simulink model "Quaternions_Method_merge_1"  (R2021b)
settings: Solver=VariableStepAuto  StartTime=0.0  StopTime=Time  FixedStep=1e-3  MinStep=1e-3  RelTol=1e-13  AbsTol=1e-8
values from neighbouring files (symbols this model uses):
  a = 8.6251e+06    (= 8625100)    [Main.m]
  c = 299792*10^3    (= 299792000)    [Main.m]
  e = 0.1195    [Main.m]
  f_mag = 5    [Main.m]
  H_0 = sqrt((g_1_0)^2 + (g_1_1)^2 + (h_1_1)^2)    [Main.m]
  i = 0.3815    [Main.m]
  MB = [2000; 0.3; 1; 0.12].*1e-2    [Main.m]
  mr = 1.2 * 0.0001    (= 0.00012)    [Main.m]
  muP = G*Mt    (= 398527110340000)    [Main.m]
  omega_0 = [om_x, om_y, om_z]    [Main.m]
  p_acc = deg2rad(5)    [Main.m]
  RD = 0.1*ones(1,10)    [Main.m]
  RS_MB = 0.5    [Main.m]
  RS_SP = 0.1    [Main.m]
  SP = [2000; 0.3; 1; 0.12].*1e-2    [Main.m]
  theta0 = 0    [Main.m]
  w_E = (2*pi)/(24*3600)    (= 7.27220521664e-05)    [Main.m]
undefined symbols (not defined in the file or in its folder): magnitude
libraries: matrix_library x10, vrlib x5, simulink_extras x1, simulink x1
(part 2 of 3)

== system Quaternions_Method_merge_1/Kinematics/Creazione Matrice A_BN/column 2 ==
  q_normalizzato : Inport
  Demux : Demux
  Gain : Gain  Gain=2
  Gain1 : Gain  Gain=2
  Mux : Mux  Inputs=3
  Product{,1..3} (4 alike) : Product
  Square{,1..3} (4 alike) : Math  Operator=square  SaturateOnIntegerOverflow=on
  Sum : Sum  Inputs=|-|+|-|+|
  Sum1 : Sum  Inputs=|+|+|
  Sum2 : Sum  Inputs=|+|-|
  Column 2 : Outport
  wires:
  Demux/4 -> [q4]
  Demux/1 -> [q1]
  q_normalizzato/1 -> Demux/1
  Demux/3 -> [q3]
  Demux/2 -> [q2]
  Mux/1 -> Column 2/1
  Gain1/1 -> Mux/3
  Product2/1 -> Sum2/1
  Product3/1 -> Sum2/2
  Sum2/1 -> Gain1/1
  Sum1/1 -> Gain/1
  [q2] -> Product/2
  [q3] -> Product1/1
  [q4] -> Product1/2
  Product/1 -> Sum1/1
  Gain/1 -> Mux/1
  [q1] -> Product/1
  Product1/1 -> Sum1/2
  Sum/1 -> Mux/2
  [q1] -> Square/1
  Square1/1 -> Sum/4
  Square3/1 -> Sum/2
  [q4] -> Square1/1
  Square2/1 -> Sum/3
  [q2] -> Square3/1
  [q3] -> Square2/1
  Square/1 -> Sum/1
  [q2] -> Product2/1
  [q3] -> Product2/2
  [q1] -> Product3/1
  [q4] -> Product3/2

== system Quaternions_Method_merge_1/Kinematics/Creazione Matrice A_BN/column 3 ==
  q_normalizzato : Inport
  Demux : Demux
  Gain : Gain  Gain=2
  Gain1 : Gain  Gain=2
  Mux : Mux  Inputs=3
  Product{,1..3} (4 alike) : Product
  Square{,1..3} (4 alike) : Math  Operator=square  SaturateOnIntegerOverflow=on
  Sum : Sum  Inputs=|-|-|+|+|
  Sum1 : Sum  Inputs=|+|-|
  Sum2 : Sum  Inputs=|+|+|
  Column 3 : Outport
  wires:
  Demux/4 -> [q4]
  Demux/1 -> [q1]
  q_normalizzato/1 -> Demux/1
  Demux/3 -> [q3]
  Demux/2 -> [q2]
  Gain/1 -> Mux/1
  Product1/1 -> Sum1/2
  [q4] -> Product1/2
  Product/1 -> Sum1/1
  Mux/1 -> Column 3/1
  [q1] -> Product/1
  Sum1/1 -> Gain/1
  [q1] -> Square/1
  Square2/1 -> Sum/3
  Square3/1 -> Sum/2
  [q4] -> Square1/1
  Square1/1 -> Sum/4
  Square/1 -> Sum/1
  Sum/1 -> Mux/3
  [q3] -> Square2/1
  [q2] -> Square3/1
  [q2] -> Product2/1
  Product3/1 -> Sum2/2
  Gain1/1 -> Mux/2
  Sum2/1 -> Gain1/1
  Product2/1 -> Sum2/1
  [q3] -> Product2/2
  [q4] -> Product3/2
  [q1] -> Product3/1
  [q3] -> Product/2
  [q2] -> Product1/1

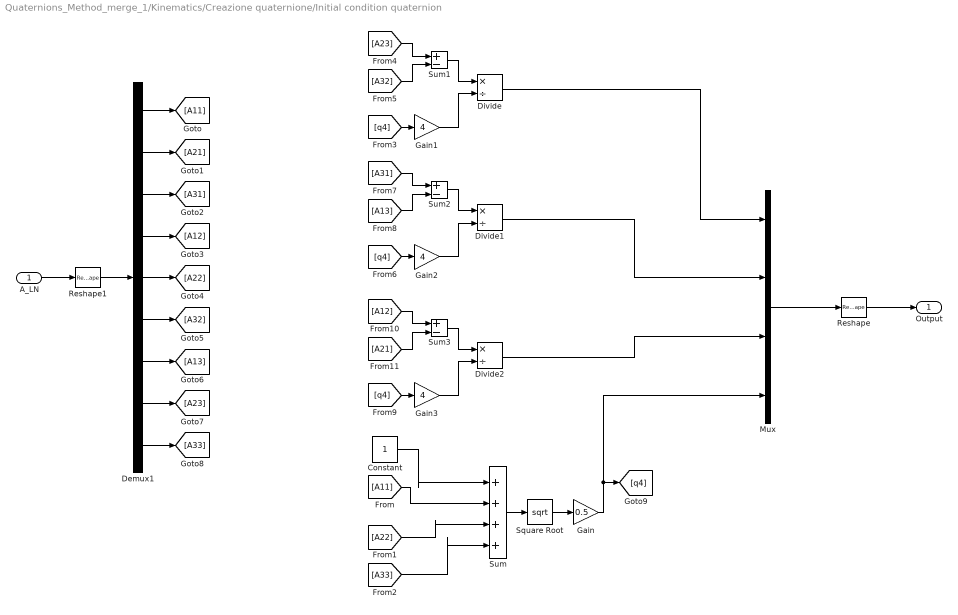
== system Quaternions_Method_merge_1/Kinematics/Creazione quaternione/Initial condition quaternion ==
  A_LN : Inport
  Constant : Constant
  Demux1 : Demux  Outputs=9
  Divide : Product  Inputs=*/
  Divide1 : Product  Inputs=*/
  Divide2 : Product  Inputs=*/
  Gain : Gain  Gain=0.5
  Gain1 : Gain  Gain=4
  Gain2 : Gain  Gain=4
  Gain3 : Gain  Gain=4
  Mux : Mux
  Reshape : Reshape  OutputDimensionality=Column vector (2-D)
  Reshape1 : Reshape  OutputDimensionality=Column vector (2-D)
  Square Root : Sqrt  SaturateOnIntegerOverflow=on
  Sum : Sum  Inputs=|+|+|+|+|
  Sum1 : Sum  Inputs=|+|-|
  Sum2 : Sum  Inputs=|+|-|
  Sum3 : Sum  Inputs=|+|-|
  Output : Outport
  wires:
  Demux1/3 -> [A31]
  Demux1/9 -> [A33]
  Demux1/1 -> [A11]
  A_LN/1 -> Reshape1/1
  Reshape1/1 -> Demux1/1
  Demux1/5 -> [A22]
  Demux1/2 -> [A21]
  Demux1/4 -> [A12]
  Demux1/6 -> [A32]
  Demux1/7 -> [A13]
  Demux1/8 -> [A23]
  Constant/1 -> Sum/1
  [A11] -> Sum/2
  [A22] -> Sum/3
  [A33] -> Sum/4
  Sum/1 -> Square Root/1
  Square Root/1 -> Gain/1
  Gain/1 -> Mux/4, [q4]
  [A23] -> Sum1/1
  [A32] -> Sum1/2
  Sum1/1 -> Divide/1
  [q4] -> Gain1/1
  Gain1/1 -> Divide/2
  Divide/1 -> Mux/1
  Divide1/1 -> Mux/2
  [A31] -> Sum2/1
  [A13] -> Sum2/2
  Sum2/1 -> Divide1/1
  [q4] -> Gain2/1
  Gain2/1 -> Divide1/2
  Divide2/1 -> Mux/3
  [A12] -> Sum3/1
  [A21] -> Sum3/2
  Sum3/1 -> Divide2/1
  [q4] -> Gain3/1
  Gain3/1 -> Divide2/2
  Mux/1 -> Reshape/1
  Reshape/1 -> Output/1

== system Quaternions_Method_merge_1/Kinematics/Creazione quaternione/Normalisation ==
  In1 : Inport
  Normalize Vector : vrlib/Utilities/Normalize Vector  maxzero=0
  Reshape : Reshape  OutputDimensionality=Column vector (2-D)
  Out1 : Outport
  wires:
  In1/1 -> Normalize Vector/1
  Normalize Vector/1 -> Reshape/1
  Reshape/1 -> Out1/1

== system Quaternions_Method_merge_1/Kinematics/Relative_Attitude/A_LN ==
  theta : Inport
  Constant : Constant  Value=i
  M1 : Subsystem
  M2 : Subsystem
  MatrixMultiply : Product  Multiplication=Matrix(*)
  A_LN : Outport
  wires:
  theta/1 -> M1/1(Input)
  M1/1(Out1) -> MatrixMultiply/1
  M2/1(Out1) -> MatrixMultiply/2
  MatrixMultiply/1 -> A_LN/1
  Constant/1 -> M2/1(ii)

== system Quaternions_Method_merge_1/Kinematics/Relative_Attitude/Orbit Propagation ==
  A_BN : Inport
  Constant : Constant  Value=muP
  Constant1 : Constant  Value=e^2
  Constant2 : Constant
  Constant3 : Constant  Value=3
  Constant4 : Constant
  Constant5 : Constant  Value=3/2
  Cos : Trigonometry  Operator=cos
  Divide : Product  Inputs=*/
  Divide1 : Product  Inputs=*/
  Divide2 : Product  Inputs=*/
  Gain : Gain  Gain=a
  Gain1 : Gain  Gain=e
  Integrator : Integrator  InitialCondition=theta0
  MatrixMultiply : Product  Multiplication=Matrix(*)
  Product : Product
  Product1 : Product
  Sqrt : Sqrt  SaturateOnIntegerOverflow=on
  Square : Math  Operator=pow  SaturateOnIntegerOverflow=on
  Square1 : Math  Operator=square  SaturateOnIntegerOverflow=on
  Square2 : Math  Operator=pow  SaturateOnIntegerOverflow=on
  Sum : Sum  Inputs=+-
  Sum1 : Sum
  vector : Subsystem
  n : Outport
  theta : Outport  Port=2
  rB : Outport  Port=3
  wires:
  Constant2/1 -> Sum/1
  Constant1/1 -> Sum/2
  Sum/1 -> Square2/1, Gain/1
  Gain/1 -> Divide/1
  Constant4/1 -> Sum1/1
  Sum1/1 -> Square1/1, Divide/2
  Gain1/1 -> Sum1/2
  Cos/1 -> Gain1/1
  Integrator/1 -> Cos/1, theta/1, vector/1(theta)  "theta"
  Divide1/1 -> Sqrt/1
  Constant/1 -> Divide1/1
  Square/1 -> Divide1/2
  Divide/1 -> Product1/1, Square/1  "R"
  Constant3/1 -> Square/2
  Sqrt/1 -> Product/1, n/1  "n"
  Square1/1 -> Product/2
  Constant5/1 -> Square2/2
  Product/1 -> Divide2/1
  Divide2/1 -> Integrator/1  "theta_dot"
  vector/1(Vector) -> Product1/2
  A_BN/1 -> MatrixMultiply/1
  Product1/1 -> MatrixMultiply/2  "rN"
  MatrixMultiply/1 -> rB/1  "rB"
  Square2/1 -> Divide2/2

== system Quaternions_Method_merge_1/Magnetometer/Magnetometer /Error Matrices ==
  A_NonOrtho : Subsystem
  A_ScaleFactor : Subsystem
  A_eps : Subsystem
  A_no : Outport
  A_sf : Outport  Port=2
  A_noise : Outport  Port=3
  wires:
  A_NonOrtho/1(A_no) -> A_no/1
  A_ScaleFactor/1(A_sf) -> A_sf/1
  A_eps/1(A_eps) -> A_noise/1

== system Quaternions_Method_merge_1/Magnetometer/Magnetometer /RC Low Pass FIlter ==
  A* : Inport
  Add : Sum  Inputs=||+||-||
  Discrete Derivative : simulink/Discrete/Discrete Derivative  gainval=10  ICPrevScaledInput=0.0  OutMin=[]  OutMax=[]  OutDataType=fixdt(1, 16)  OutScaling=2^-10  DoSatur=off
  A*_filtered : Outport
  wires:
  A*/1 -> Add/1
  Add/1 -> Discrete Derivative/1, A*_filtered/1
  Discrete Derivative/1 -> Add/2

== system Quaternions_Method_merge_1/Magnetometer/Magnetometer /orthonormalization step 1 ==
  A*(t) : Inport
  Gain : Gain  Gain=3/2
  Gain1 : Gain  Gain=1/2
  Matrix Multiply : Product  Inputs=3  Multiplication=Matrix(*)
  Sum : Sum  Inputs=-+
  Transpose : Math  Operator=transpose  SaturateOnIntegerOverflow=on
  A_BN*_filtered : Outport
  wires:
  A*(t)/1 -> Transpose/1, Gain1/1, Matrix Multiply/1, Gain/1
  Sum/1 -> A_BN*_filtered/1
  Gain/1 -> Sum/2
  Transpose/1 -> Matrix Multiply/2
  Gain1/1 -> Matrix Multiply/3
  Matrix Multiply/1 -> Sum/1

== system Quaternions_Method_merge_1/Magnetometer/Magnetometer /orthonormalization step 2 ==
  A*(t) : Inport
  Gain : Gain  Gain=3/2
  Gain1 : Gain  Gain=1/2
  Matrix Multiply : Product  Inputs=3  Multiplication=Matrix(*)
  Sum : Sum  Inputs=-+
  Transpose : Math  Operator=transpose  SaturateOnIntegerOverflow=on
  A_BN*_filtered : Outport
  wires:
  Matrix Multiply/1 -> Sum/1
  Gain1/1 -> Matrix Multiply/3
  Transpose/1 -> Matrix Multiply/2
  Gain/1 -> Sum/2
  Sum/1 -> A_BN*_filtered/1
  A*(t)/1 -> Gain/1, Matrix Multiply/1, Gain1/1, Transpose/1

== system Quaternions_Method_merge_1/Magnetometer/Magnetometer /orthonormalization step 3 ==
  A*(t) : Inport
  Gain : Gain  Gain=3/2
  Gain1 : Gain  Gain=1/2
  Matrix Multiply : Product  Inputs=3  Multiplication=Matrix(*)
  Sum : Sum  Inputs=-+
  Transpose : Math  Operator=transpose  SaturateOnIntegerOverflow=on
  A_BN*_filtered : Outport
  wires:
  A*(t)/1 -> Transpose/1, Gain1/1, Matrix Multiply/1, Gain/1
  Sum/1 -> A_BN*_filtered/1
  Gain/1 -> Sum/2
  Transpose/1 -> Matrix Multiply/2
  Gain1/1 -> Matrix Multiply/3
  Matrix Multiply/1 -> Sum/1

== system Quaternions_Method_merge_1/Magnetometer/b_B computation/Saturation ==
  b_B : Inport
  Constant : Constant  Value=mr
  Dot Product : DotProduct  InputSameDT=on  OutDataTypeStr=Inherit: Inherit via internal rule
  If : If  NumInputs=2  IfExpression=u1 < mr
  If Action Subsystem : Subsystem  TreatAsAtomicUnit=on
  If Action Subsystem1 : Subsystem  TreatAsAtomicUnit=on
  Merge : Merge
  Square Root : Sqrt  SaturateOnIntegerOverflow=on
  b_B saturated : Outport
  wires:
  b_B/1 -> If Action Subsystem1/2(In2), If Action Subsystem/1(In1), Dot Product/2, Dot Product/1
  Dot Product/1 -> Square Root/1
  If Action Subsystem/1(b_B) -> Merge/1
  If/1 -> If Action Subsystem/Action
  If Action Subsystem1/1(Out1) -> Merge/2
  If/2 -> If Action Subsystem1/Action
  Square Root/1 -> If/1
  Constant/1 -> If Action Subsystem1/1(In1), If/2
  Merge/1 -> b_B saturated/1

== system Quaternions_Method_merge_1/Enviroment/Magnetic torque /Magnetic torque in body frame/Definition of m vector ==
  Clock : Clock
  Constant : Constant  Value=eps
  Constant1 : Constant  Value=w_E
  Mux : Mux  Inputs=3
  Product : Product
  Product1 : Product
  Product2 : Product
  Reshape : Reshape  OutputDimensionality=Column vector (2-D)
  Trigonometric Function : Trigonometry
  Trigonometric Function1 : Trigonometry  Operator=cos
  Trigonometric Function2 : Trigonometry  Operator=cos
  Trigonometric Function3 : Trigonometry
  m_vect : Outport
  wires:
  Constant1/1 -> Product/1
  Clock/1 -> Product/2
  Constant/1 -> Trigonometric Function2/1, Trigonometric Function/1
  Product/1 -> Trigonometric Function3/1, Trigonometric Function1/1
  Trigonometric Function/1 -> Product2/1, Product1/1
  Trigonometric Function1/1 -> Product1/2
  Trigonometric Function3/1 -> Product2/2
  Product1/1 -> Mux/1
  Product2/1 -> Mux/2
  Trigonometric Function2/1 -> Mux/3
  Mux/1 -> Reshape/1
  Reshape/1 -> m_vect/1

== system Quaternions_Method_merge_1/Enviroment/Solar Radiation Perturbation/Force/creation of the areas of the S//C ==
  note: creation of areas of MB:
      | a=lato corto su asse x del BF; b=lato lungo lungo asse y del BF; h = spessore lungo asse z del BF
  MB : Inport
  Demux : Demux
  Product1 : Product
  Product2 : Product
  Product4 : Product
  Terminator : Terminator
  a*b_1 : Outport
  a*b_2 : Outport  Port=2
  a*h_1 : Outport  Port=3
  a*h_2 : Outport  Port=4
  b*h_1 : Outport  Port=5
  b*h_2 : Outport  Port=6
  wires:
  Demux/4 -> Product4/1, Product2/2
  Demux/3 -> Product1/2, Product4/2
  Demux/2 -> Product1/1, Product2/1
  Product1/1 -> a*b_2/1, a*b_1/1  "a*b"
  Product2/1 -> a*h_1/1, a*h_2/1  "a*h"
  Product4/1 -> b*h_2/1, b*h_1/1  "b*h"
  MB/1 -> Demux/1
  Demux/1 -> Terminator/1

== system Quaternions_Method_merge_1/Enviroment/Solar Radiation Perturbation/Sum forces/determine highlighted area ==
  note: matrice che ha per colonne i vettori distanza tra il CM del MB e i centri geom delle aree illuminate dal sole
  MB : Inport
  A_MB : Inport  Port=2
  prodscal_MB(tra norm e sun direction) : Inport  Port=3
  Demux1 : Demux  Outputs=6
  Demux2 : Demux  Outputs=6
  If : If  NumInputs=2  IfExpression=u1>0  ElseIfExpressions=u2>0
  If Action Subsystem : Subsystem  TreatAsAtomicUnit=on
  If Action Subsystem1 : Subsystem  TreatAsAtomicUnit=on
  If Action Subsystem2 : Subsystem  TreatAsAtomicUnit=on
  If Action Subsystem3 : Subsystem  TreatAsAtomicUnit=on
  If Action Subsystem4 : Subsystem  TreatAsAtomicUnit=on
  If Action Subsystem5 : Subsystem  TreatAsAtomicUnit=on
  If Action Subsystem6 : Subsystem  TreatAsAtomicUnit=on
  If Action Subsystem7 : Subsystem  TreatAsAtomicUnit=on
  If Action Subsystem8 : Subsystem  TreatAsAtomicUnit=on
  If1 : If  NumInputs=2  IfExpression=u1>0  ElseIfExpressions=u2>0
  If2 : If  NumInputs=2  IfExpression=u1>0  ElseIfExpressions=u2>0
  Merge : Merge  Inputs=3
  Merge1 : Merge  Inputs=3
  Merge2 : Merge  Inputs=3
  Mux : Mux  Inputs=3
  Product{10..15} (6 alike) : Product
  Reshape : Reshape  OutputDimensionality=Column vector (2-D)
  Reshape1 : Reshape  OutputDimensionality=Column vector (2-D)
  "creazione della matrice che ha per colonne i vettori distanza tra il CM del MB e i centri geom delle aree illuminate dal sole " : Subsystem
  distance matrix : Outport
  wires:
  Reshape/1 -> Demux2/1
  prodscal_MB(tra norm e sun direction)/1 -> Reshape/1
  Demux2/1 -> Product15/2  "x"
  Demux2/2 -> Product13/2  "y"
  Demux2/3 -> Product12/2  "z"
  Demux2/4 -> Product11/2  "-x"
  Demux2/5 -> Product10/2  "-y"
  Demux2/6 -> Product14/2  "-z"
  Demux1/1 -> Product12/1
  Mux/1 -> Reshape1/1
  Product15/1 -> If Action Subsystem/1(In1), If/1  "x"
  If/1 -> If Action Subsystem/Action
  Reshape1/1 -> "creazione della matrice che ha per colonne i vettori distanza tra il CM del MB e i centri geom delle aree illuminate dal sole "/2(A_vect)  "Areas_vect = vettore contenente le aree nelle direzioni x, y, z, -x, -y, -z"
  "creazione della matrice che ha per colonne i vettori distanza tra il CM del MB e i centri geom delle aree illuminate dal sole "/1(distance matrix) -> distance matrix/1
  A_MB/1 -> Demux1/1
  Demux1/2 -> Product14/1
  Demux1/3 -> Product13/1
  Demux1/4 -> Product10/1
  Demux1/5 -> Product15/1
  Demux1/6 -> Product11/1
  If/2 -> If Action Subsystem1/Action
  Product11/1 -> If Action Subsystem1/1(In1), If/2  "-x"
  If1/2 -> If Action Subsystem4/Action
  If1/3 -> If Action Subsystem5/Action
  If1/1 -> If Action Subsystem3/Action
  Product10/1 -> If Action Subsystem4/1(In1), If1/2  "-y"
  Product13/1 -> If Action Subsystem3/1(In1), If1/1  "y"
  If2/2 -> If Action Subsystem7/Action
  If2/3 -> If Action Subsystem8/Action
  If2/1 -> If Action Subsystem6/Action
  Product12/1 -> If Action Subsystem6/1(In1), If2/1  "z"
  Product14/1 -> If Action Subsystem7/1(In1), If2/2  "-z"
  Merge/1 -> Mux/2
  Merge2/1 -> Mux/3
  Merge1/1 -> Mux/1
  If Action Subsystem8/1(Out1) -> Merge2/3
  If Action Subsystem7/1(Out1) -> Merge2/2
  If Action Subsystem6/1(Out1) -> Merge2/1
  If Action Subsystem5/1(Out1) -> Merge/3
  If Action Subsystem4/1(Out1) -> Merge/2
  MB/1 -> "creazione della matrice che ha per colonne i vettori distanza tra il CM del MB e i centri geom delle aree illuminate dal sole "/1(MB)
  If Action Subsystem/1(Out1) -> Merge1/1
  If Action Subsystem1/1(Out1) -> Merge1/2
  If/3 -> If Action Subsystem2/Action
  If Action Subsystem2/1(Out1) -> Merge1/3
  If Action Subsystem3/1(Out1) -> Merge/1

== system Quaternions_Method_merge_1/Enviroment/Solar Radiation Perturbation/Sum forces/determine highlighted area1 ==
  prodscal_SP(tra norm e sun direction) : Inport
  Demux2 : Demux
  If : If  NumInputs=2  IfExpression=u1>0  ElseIfExpressions=u2>0
  If Action Subsystem : Subsystem  TreatAsAtomicUnit=on
  If Action Subsystem1 : Subsystem  TreatAsAtomicUnit=on
  If Action Subsystem2 : Subsystem  TreatAsAtomicUnit=on
  If Action Subsystem3 : Subsystem  TreatAsAtomicUnit=on
  If Action Subsystem4 : Subsystem  TreatAsAtomicUnit=on
  If Action Subsystem5 : Subsystem  TreatAsAtomicUnit=on
  If1 : If  NumInputs=2  IfExpression=u1>0  ElseIfExpressions=u2>0
  Merge : Merge  Inputs=3
  Merge1 : Merge  Inputs=3
  Mux : Mux  Inputs=2
  Reshape : Reshape  OutputDimensionality=Column vector (2-D)
  Reshape1 : Reshape  OutputDimensionality=Column vector (2-D)
  face illuminated : Outport
  wires:
  If Action Subsystem2/1(Out1) -> Merge/3
  If/3 -> If Action Subsystem2/Action
  Merge/1 -> Mux/1
  Demux2/1 -> If/1  "y_1"
  Mux/1 -> Reshape1/1
  Demux2/2 -> If/2  "-y_1"
  prodscal_SP(tra norm e sun direction)/1 -> Reshape/1
  Reshape/1 -> Demux2/1
  Demux2/3 -> If1/1  "y_2"
  Demux2/4 -> If1/2  "-y_2"
  Merge1/1 -> Mux/2
  Reshape1/1 -> face illuminated/1
  If/1 -> If Action Subsystem/Action
  If Action Subsystem/1(Out1) -> Merge/1
  If/2 -> If Action Subsystem1/Action
  If Action Subsystem1/1(Out1) -> Merge/2
  If Action Subsystem4/1(Out1) -> Merge1/2
  If1/2 -> If Action Subsystem4/Action
  If1/1 -> If Action Subsystem3/Action
  If1/3 -> If Action Subsystem5/Action
  If Action Subsystem5/1(Out1) -> Merge1/3
  If Action Subsystem3/1(Out1) -> Merge1/1

== system Quaternions_Method_merge_1/Kinematics/Relative_Attitude/A_LN/M1 ==
  Input : Inport
  Constant{1..2,4..5} (4 alike) : Constant  Value=0
  Constant3 : Constant
  Cos : Trigonometry  Operator=cos
  Cos1 : Trigonometry
  Cos2 : Trigonometry  Operator=cos
  Cos3 : Trigonometry
  Matrix Concatenate : Concatenate  NumInputs=3  Mode=Multidimensional array  ConcatenateDimension=2
  Multiply : Gain  Gain=-1
  Mux : Mux  Inputs=3
  Mux1 : Mux  Inputs=3
  Mux2 : Mux  Inputs=3
  Reshape : Reshape  OutputDimensionality=Column vector (2-D)
  Reshape1 : Reshape  OutputDimensionality=Column vector (2-D)
  Reshape2 : Reshape  OutputDimensionality=Column vector (2-D)
  Out1 : Outport
  wires:
  Multiply/1 -> Mux/2
  Cos/1 -> Mux/1
  Constant1/1 -> Mux/3
  Constant2/1 -> Mux1/3
  Input/1 -> Cos/1, Cos1/1, Cos3/1, Cos2/1
  Matrix Concatenate/1 -> Out1/1
  Cos3/1 -> Mux1/1
  Constant5/1 -> Mux2/1
  Cos2/1 -> Mux1/2
  Constant3/1 -> Mux2/3
  Constant4/1 -> Mux2/2
  Cos1/1 -> Multiply/1
  Mux/1 -> Reshape/1
  Reshape/1 -> Matrix Concatenate/1
  Reshape1/1 -> Matrix Concatenate/2
  Mux1/1 -> Reshape1/1
  Mux2/1 -> Reshape2/1
  Reshape2/1 -> Matrix Concatenate/3

== system Quaternions_Method_merge_1/Kinematics/Relative_Attitude/A_LN/M2 ==
  ii : Inport
  Constant{1..4} (4 alike) : Constant  Value=0
  Constant5 : Constant
  Cos : Trigonometry  Operator=cos
  Cos1 : Trigonometry
  Cos2 : Trigonometry  Operator=cos
  Cos3 : Trigonometry
  Matrix Concatenate : Concatenate  NumInputs=3  Mode=Multidimensional array  ConcatenateDimension=2
  Multiply : Gain  Gain=-1
  Mux : Mux  Inputs=3
  Mux1 : Mux  Inputs=3
  Mux2 : Mux  Inputs=3
  Reshape : Reshape  OutputDimensionality=Column vector (2-D)
  Reshape1 : Reshape  OutputDimensionality=Column vector (2-D)
  Reshape2 : Reshape  OutputDimensionality=Column vector (2-D)
  Out1 : Outport
  wires:
  Matrix Concatenate/1 -> Out1/1
  Constant5/1 -> Mux2/1
  Constant3/1 -> Mux2/3
  Constant4/1 -> Mux2/2
  Cos1/1 -> Multiply/1
  Constant1/1 -> Mux/1
  Cos/1 -> Mux/2
  Multiply/1 -> Mux/3
  Constant2/1 -> Mux1/1
  Cos3/1 -> Mux1/2
  Cos2/1 -> Mux1/3
  ii/1 -> Cos2/1, Cos/1, Cos1/1, Cos3/1
  Mux2/1 -> Reshape/1
  Reshape/1 -> Matrix Concatenate/1
  Mux/1 -> Reshape1/1
  Reshape1/1 -> Matrix Concatenate/2
  Reshape2/1 -> Matrix Concatenate/3
  Mux1/1 -> Reshape2/1

== system Quaternions_Method_merge_1/Kinematics/Relative_Attitude/Orbit Propagation/vector ==
  theta : Inport
  Constant : Constant  Value=i
  Cos : Trigonometry  Operator=cos
  Cos1 : Trigonometry
  Cos2 : Trigonometry  Operator=cos
  Cos3 : Trigonometry
  Cos4 : Trigonometry
  Mux : Mux  Inputs=3
  Product : Product
  Product1 : Product
  Vector : Outport
  wires:
  Mux/1 -> Vector/1
  Cos/1 -> Mux/1
  Cos1/1 -> Product/1
  Cos2/1 -> Product/2
  Product/1 -> Mux/2
  Cos4/1 -> Product1/2
  Product1/1 -> Mux/3
  Cos3/1 -> Product1/1
  theta/1 -> Cos3/1, Cos1/1, Cos/1
  Constant/1 -> Cos4/1, Cos2/1

== system Quaternions_Method_merge_1/Magnetometer/Magnetometer /Error Matrices/A_NonOrtho ==
  Constant : Constant
  Constant1 : Constant  Value=0
  Constant2 : Constant  Value=0
  Constant3 : Constant  Value=-0.04
  Constant4 : Constant
  Constant5 : Constant  Value=0
  Constant6 : Constant  Value=0.02
  Constant7 : Constant  Value=0.01
  Constant8 : Constant
  Reshape : Reshape  OutputDimensionality=Customize  OutputDimensions=[3,3]
  Vector Concatenate : Concatenate  NumInputs=9
  A_no : Outport
  wires:
  [A31] -> Vector Concatenate/3
  [A12] -> Vector Concatenate/4
  [A21] -> Vector Concatenate/2
  [A33] -> Vector Concatenate/9
  [A32] -> Vector Concatenate/6
  [A22] -> Vector Concatenate/5
  [A13] -> Vector Concatenate/7
  [A23] -> Vector Concatenate/8
  [A11] -> Vector Concatenate/1
  Vector Concatenate/1 -> Reshape/1
  Reshape/1 -> A_no/1
  Constant/1 -> [A11]
  Constant1/1 -> [A21]
  Constant2/1 -> [A31]
  Constant3/1 -> [A12]
  Constant4/1 -> [A22]
  Constant5/1 -> [A32]
  Constant6/1 -> [A13]
  Constant7/1 -> [A23]
  Constant8/1 -> [A33]

== system Quaternions_Method_merge_1/Magnetometer/Magnetometer /Error Matrices/A_ScaleFactor ==
  Constant : Constant  Value=1.08
  Constant{1..2,4..7} (6 alike) : Constant  Value=0
  Constant3 : Constant  Value=0.95
  Constant8 : Constant  Value=1.10
  Reshape : Reshape  OutputDimensionality=Customize  OutputDimensions=[3,3]
  Vector Concatenate : Concatenate  NumInputs=9
  A_sf : Outport
  wires:
  [A31] -> Vector Concatenate/3
  [A12] -> Vector Concatenate/4
  [A21] -> Vector Concatenate/2
  [A33] -> Vector Concatenate/9
  [A32] -> Vector Concatenate/6
  [A22] -> Vector Concatenate/5
  [A13] -> Vector Concatenate/7
  [A23] -> Vector Concatenate/8
  [A11] -> Vector Concatenate/1
  Vector Concatenate/1 -> Reshape/1
  Reshape/1 -> A_sf/1
  Constant/1 -> [A11]
  Constant1/1 -> [A21]
  Constant2/1 -> [A31]
  Constant4/1 -> [A12]
  Constant3/1 -> [A22]
  Constant5/1 -> [A32]
  Constant6/1 -> [A13]
  Constant7/1 -> [A23]
  Constant8/1 -> [A33]

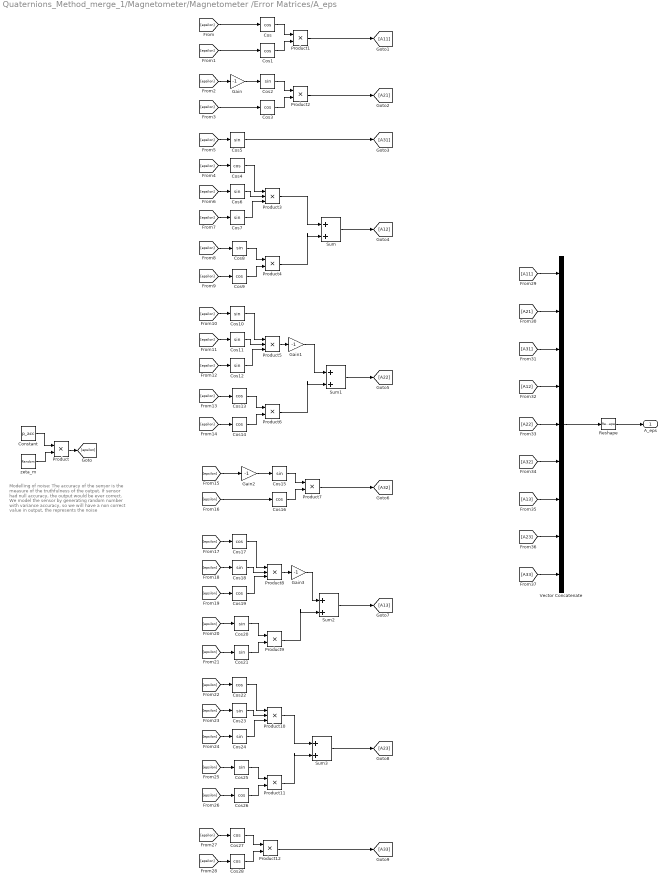
== system Quaternions_Method_merge_1/Magnetometer/Magnetometer /Error Matrices/A_eps ==
  note: Modelling of noise: The accuracy of the sensor
      | is the measure of the truthfulness of the output.
      | If sensor had null accuracy, the output would be
      | ever correct. We model the  sensor by generating
      | random number with variance accuracy, so we
      | will have a non correct value in output, the
      | represents the noise
  Constant : Constant  Value=p_acc
  Cos{,1,3..4,9,13..14,16..17,19,22,26..28} (14 alike) : Trigonometry  Operator=cos
  Cos{2,5..8,10..12,15,18,20..21,23..25} (15 alike) : Trigonometry
  Gain{,1..3} (4 alike) : Gain  Gain=-1
  Product{,1..2,4,6..7,9,11..12} (9 alike) : Product
  Product{3,5,8,10} (4 alike) : Product  Inputs=3
  Reshape : Reshape  OutputDimensionality=Customize  OutputDimensions=[3,3]
  Sum{,1..3} (4 alike) : Sum  Inputs=|+|+|
  Vector Concatenate : Concatenate  NumInputs=9
  zeta_m : RandomNumber  Variance=p_acc  Seed=1  SampleTime=1/f_mag
  A_eps : Outport
  wires:
  Reshape/1 -> A_eps/1
  Vector Concatenate/1 -> Reshape/1
  Constant/1 -> Product/1
  zeta_m/1 -> Product/2
  Product/1 -> [epsilon]
  [epsilon] -> Cos/1
  [epsilon] -> Cos1/1
  Cos/1 -> Product1/1
  Cos1/1 -> Product1/2
  Product1/1 -> [A11]
  Cos2/1 -> Product2/1
  Cos3/1 -> Product2/2
  [epsilon] -> Cos3/1
  Product2/1 -> [A21]
  [epsilon] -> Gain/1
  Gain/1 -> Cos2/1
  [epsilon] -> Cos5/1
  Cos5/1 -> [A31]
  Cos4/1 -> Product3/1
  Cos6/1 -> Product3/2
  [epsilon] -> Cos4/1
  [epsilon] -> Cos6/1
  Product3/1 -> Sum/1
  [epsilon] -> Cos7/1
  Cos7/1 -> Product3/3
  [epsilon] -> Cos8/1
  Product4/1 -> Sum/2
  [epsilon] -> Cos9/1
  Cos9/1 -> Product4/2
  Cos8/1 -> Product4/1
  Sum/1 -> [A12]
  [epsilon] -> Cos11/1
  [epsilon] -> Cos10/1
  Cos11/1 -> Product5/2
  Cos10/1 -> Product5/1
  [epsilon] -> Cos13/1
  Sum1/1 -> [A22]
  Cos13/1 -> Product6/1
  [epsilon] -> Cos14/1
  Cos12/1 -> Product5/3
  Cos14/1 -> Product6/2
  Product6/1 -> Sum1/2
  [epsilon] -> Cos12/1
  Product5/1 -> Gain1/1
  Gain1/1 -> Sum1/1
  Gain2/1 -> Cos15/1
  [epsilon] -> Gain2/1
  Product7/1 -> [A32]
  Cos16/1 -> Product7/2
  Cos15/1 -> Product7/1
  [epsilon] -> Cos16/1
  Gain3/1 -> Sum2/1
  Product8/1 -> Gain3/1
  Cos18/1 -> Product8/2
  [epsilon] -> Cos18/1
  Sum2/1 -> [A13]
  Cos20/1 -> Product9/1
  Cos17/1 -> Product8/1
  [epsilon] -> Cos19/1
  Cos19/1 -> Product8/3
  Product9/1 -> Sum2/2
  [epsilon] -> Cos17/1
  Cos21/1 -> Product9/2
  [epsilon] -> Cos20/1
  [epsilon] -> Cos21/1
  [epsilon] -> Cos23/1
  [epsilon] -> Cos22/1
  Cos23/1 -> Product10/2
  Cos22/1 -> Product10/1
  [epsilon] -> Cos25/1
  Sum3/1 -> [A23]
  Cos25/1 -> Product11/1
  [epsilon] -> Cos26/1
  Product10/1 -> Sum3/1
  Cos24/1 -> Product10/3
  Cos26/1 -> Product11/2
  Product11/1 -> Sum3/2
  [epsilon] -> Cos24/1
  Cos27/1 -> Product12/1
  Cos28/1 -> Product12/2
  [epsilon] -> Cos27/1
  [epsilon] -> Cos28/1
  Product12/1 -> [A33]
  [A11] -> Vector Concatenate/1
  [A21] -> Vector Concatenate/2
  [A31] -> Vector Concatenate/3
  [A12] -> Vector Concatenate/4
  [A22] -> Vector Concatenate/5
  [A32] -> Vector Concatenate/6
  [A13] -> Vector Concatenate/7
  [A23] -> Vector Concatenate/8
  [A33] -> Vector Concatenate/9

== system Quaternions_Method_merge_1/Magnetometer/b_B computation/Saturation/If Action Subsystem ==
  In1 : Inport
  Action Port : ActionPort  ActionPortLabel=if(u1 < mr)
  b_B : Outport
  wires:
  In1/1 -> b_B/1

== system Quaternions_Method_merge_1/Magnetometer/b_B computation/Saturation/If Action Subsystem1 ==
  In1 : Inport
  In2 : Inport  Port=2
  Action Port : ActionPort  ActionPortLabel=else
  Normalize Vector : vrlib/Utilities/Normalize Vector  maxzero=0
  Product : Product
  Out1 : Outport
  wires:
  In2/1 -> Normalize Vector/1
  Product/1 -> Out1/1
  In1/1 -> Product/1
  Normalize Vector/1 -> Product/2

== system Quaternions_Method_merge_1/Enviroment/Solar Radiation Perturbation/Sum forces/determine highlighted area/If Action Subsystem ==
  In1 : Inport
  Action Port : ActionPort  ActionPortLabel=if(u1>0 )
  Out1 : Outport
  wires:
  In1/1 -> Out1/1

== system Quaternions_Method_merge_1/Enviroment/Solar Radiation Perturbation/Sum forces/determine highlighted area/If Action Subsystem1 ==
  In1 : Inport
  Action Port : ActionPort  ActionPortLabel=elseif(u2>0)
  Out1 : Outport
  wires:
  In1/1 -> Out1/1

== system Quaternions_Method_merge_1/Enviroment/Solar Radiation Perturbation/Sum forces/determine highlighted area/If Action Subsystem2 ==
  Action Port : ActionPort  ActionPortLabel=else
  Constant : Constant  Value=0
  Out1 : Outport
  wires:
  Constant/1 -> Out1/1

== system Quaternions_Method_merge_1/Enviroment/Solar Radiation Perturbation/Sum forces/determine highlighted area/If Action Subsystem3 ==
  In1 : Inport
  Action Port : ActionPort  ActionPortLabel=if(u1>0 )
  Out1 : Outport
  wires:
  In1/1 -> Out1/1

== system Quaternions_Method_merge_1/Enviroment/Solar Radiation Perturbation/Sum forces/determine highlighted area/If Action Subsystem4 ==
  In1 : Inport
  Action Port : ActionPort  ActionPortLabel=elseif(u2>0)
  Out1 : Outport
  wires:
  In1/1 -> Out1/1

== system Quaternions_Method_merge_1/Enviroment/Solar Radiation Perturbation/Sum forces/determine highlighted area/If Action Subsystem5 ==
  Action Port : ActionPort  ActionPortLabel=else
  Constant : Constant  Value=0
  Out1 : Outport
  wires:
  Constant/1 -> Out1/1

== system Quaternions_Method_merge_1/Enviroment/Solar Radiation Perturbation/Sum forces/determine highlighted area/If Action Subsystem6 ==
  In1 : Inport
  Action Port : ActionPort  ActionPortLabel=if(u1>0 )
  Out1 : Outport
  wires:
  In1/1 -> Out1/1

== system Quaternions_Method_merge_1/Enviroment/Solar Radiation Perturbation/Sum forces/determine highlighted area/If Action Subsystem7 ==
  In1 : Inport
  Action Port : ActionPort  ActionPortLabel=elseif(u2>0)
  Out1 : Outport
  wires:
  In1/1 -> Out1/1

== system Quaternions_Method_merge_1/Enviroment/Solar Radiation Perturbation/Sum forces/determine highlighted area/If Action Subsystem8 ==
  Action Port : ActionPort  ActionPortLabel=else
  Constant : Constant  Value=0
  Out1 : Outport
  wires:
  Constant/1 -> Out1/1

== system Quaternions_Method_merge_1/Enviroment/Solar Radiation Perturbation/Sum forces/determine highlighted area/creazione della matrice che ha per colonne i vettori distanza tra il CM del MB e i centri geom delle aree illuminate dal sole  ==
  note: creo il vettore somma che ha per colonna i raggi vettori che collegano il CM del MB con i centri illuminati delle facce nel caso che il sole sia nelle 4 posizioni.
  MB : Inport
  A_vect : Inport  Port=2
  Gain : Gain  Gain=-1
  Gain1 : Gain  Gain=-1
  Gain2 : Gain  Gain=-1
  Reshape : Reshape  OutputDimensionality=Customize  OutputDimensions=[3,6]
  Transpose : Math  Operator=transpose  SaturateOnIntegerOverflow=on
  Vector Concatenate : Concatenate  NumInputs=6
  creazione raggi vettore tra CM MB e centro facce illuminate della faccia che ha come normale l'asse i : Subsystem
  creazione raggi vettore tra CM MB e centro facce illuminate della faccia che ha come normale l'asse j : Subsystem
  creazione raggi vettore tra CM MB e centro facce illuminate della faccia che ha come normale l'asse k : Subsystem
  distance matrix : Outport
  tag scope: A_vect=global
  wires:
  creazione raggi vettore tra CM MB e centro facce illuminate della faccia che ha come normale l'asse k/1(Out1) -> Gain/1, Vector Concatenate/1
  Vector Concatenate/1 -> Reshape/1  "Areas k,-k,i,-i,j,-j"
  [S_B] -> creazione raggi vettore tra CM MB e centro facce illuminate della faccia che ha come normale l'asse k/1(S_B)
  [S_B] -> creazione raggi vettore tra CM MB e centro facce illuminate della faccia che ha come normale l'asse i/1(S_B)
  [S_B] -> creazione raggi vettore tra CM MB e centro facce illuminate della faccia che ha come normale l'asse j/1(S_B)
  A_vect/1 -> [A_vect]
  Gain/1 -> Vector Concatenate/2
  creazione raggi vettore tra CM MB e centro facce illuminate della faccia che ha come normale l'asse i/1(Out1) -> Gain1/1, Vector Concatenate/3
  Gain1/1 -> Vector Concatenate/4
  Gain2/1 -> Vector Concatenate/6
  creazione raggi vettore tra CM MB e centro facce illuminate della faccia che ha come normale l'asse j/1(Out1) -> Gain2/1, Vector Concatenate/5
  Reshape/1 -> Transpose/1
  Transpose/1 -> distance matrix/1
  MB/1 -> [MB]
  [MB] -> creazione raggi vettore tra CM MB e centro facce illuminate della faccia che ha come normale l'asse k/2(MB)
  [MB] -> creazione raggi vettore tra CM MB e centro facce illuminate della faccia che ha come normale l'asse i/2(MB)
  [MB] -> creazione raggi vettore tra CM MB e centro facce illuminate della faccia che ha come normale l'asse j/2(MB)

== system Quaternions_Method_merge_1/Enviroment/Solar Radiation Perturbation/Sum forces/determine highlighted area1/If Action Subsystem ==
  Action Port : ActionPort  ActionPortLabel=if(u1>0 )
  Constant : Constant  Value=[1;0]
  Out1 : Outport
  wires:
  Constant/1 -> Out1/1

== system Quaternions_Method_merge_1/Enviroment/Solar Radiation Perturbation/Sum forces/determine highlighted area1/If Action Subsystem1 ==
  Action Port : ActionPort  ActionPortLabel=elseif(u2>0)
  Constant : Constant  Value=[0;1]
  Out1 : Outport
  wires:
  Constant/1 -> Out1/1

== system Quaternions_Method_merge_1/Enviroment/Solar Radiation Perturbation/Sum forces/determine highlighted area1/If Action Subsystem2 ==
  Action Port : ActionPort  ActionPortLabel=else
  Constant : Constant  Value=[0;0]
  Out1 : Outport
  wires:
  Constant/1 -> Out1/1

== system Quaternions_Method_merge_1/Enviroment/Solar Radiation Perturbation/Sum forces/determine highlighted area1/If Action Subsystem3 ==
  Action Port : ActionPort  ActionPortLabel=if(u1>0 )
  Constant : Constant  Value=[1;0]
  Out1 : Outport
  wires:
  Constant/1 -> Out1/1

== system Quaternions_Method_merge_1/Enviroment/Solar Radiation Perturbation/Sum forces/determine highlighted area1/If Action Subsystem4 ==
  Action Port : ActionPort  ActionPortLabel=elseif(u2>0)
  Constant : Constant  Value=[0;1]
  Out1 : Outport
  wires:
  Constant/1 -> Out1/1

== system Quaternions_Method_merge_1/Enviroment/Solar Radiation Perturbation/Sum forces/determine highlighted area1/If Action Subsystem5 ==
  Action Port : ActionPort  ActionPortLabel=else
  Constant : Constant  Value=[0;0]
  Out1 : Outport
  wires:
  Constant/1 -> Out1/1

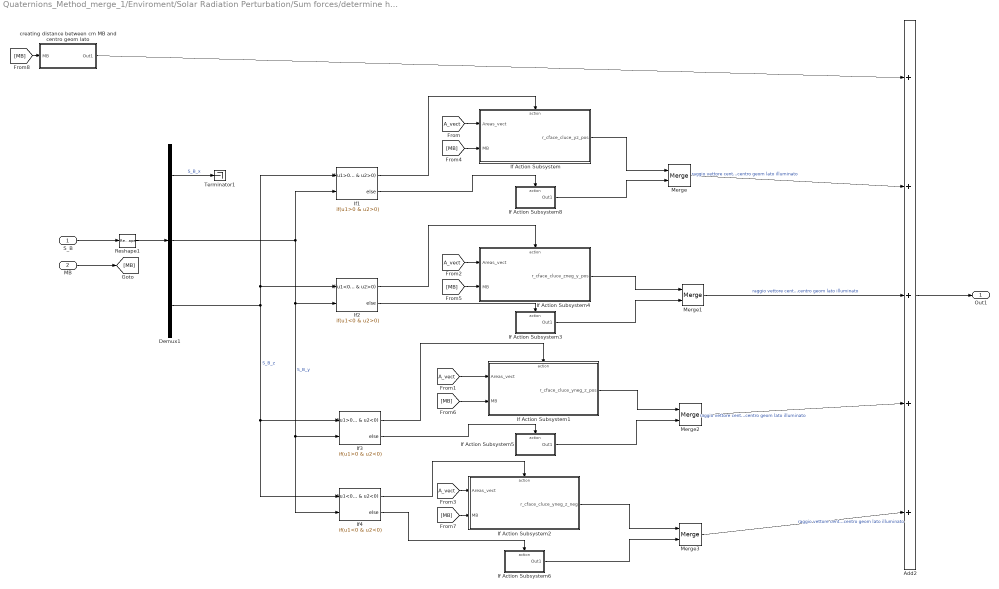
== system Quaternions_Method_merge_1/Enviroment/Solar Radiation Perturbation/Sum forces/determine highlighted area/creazione della matrice che ha per colonne i vettori distanza tra il CM del MB e i centri geom delle aree illuminate dal sole /creazione raggi vettore tra CM MB e centro facce illuminate della faccia che ha come normale l'asse i ==
  S_B : Inport
  MB : Inport  Port=2
  Add2 : Sum  Inputs=+|+|+|+|+
  Demux1 : Demux  Outputs=3
  If Action Subsystem : Subsystem  TreatAsAtomicUnit=on
  If Action Subsystem1 : Subsystem  TreatAsAtomicUnit=on
  If Action Subsystem2 : Subsystem  TreatAsAtomicUnit=on
  If Action Subsystem3 : Subsystem  TreatAsAtomicUnit=on
  If Action Subsystem4 : Subsystem  TreatAsAtomicUnit=on
  If Action Subsystem5 : Subsystem  TreatAsAtomicUnit=on
  If Action Subsystem6 : Subsystem  TreatAsAtomicUnit=on
  If Action Subsystem8 : Subsystem  TreatAsAtomicUnit=on
  If1 : If  NumInputs=2  IfExpression=u1>0 & u2>0
  If2 : If  NumInputs=2  IfExpression=u1<0 & u2>0
  If3 : If  NumInputs=2  IfExpression=u1>0 & u2<0
  If4 : If  NumInputs=2  IfExpression=u1<0 & u2<0
  Merge{,1..3} (4 alike) : Merge
  Reshape1 : Reshape  OutputDimensionality=Column vector (2-D)
  Terminator1 : Terminator
  creating distance between cm MB and centro geom lato : Subsystem
  Out1 : Outport
  wires:
  [A_vect] -> If Action Subsystem2/1(Areas_vect)
  [A_vect] -> If Action Subsystem1/1(Areas_vect)
  [A_vect] -> If Action Subsystem4/1(Areas_vect)
  Add2/1 -> Out1/1
  Merge3/1 -> Add2/5  "raggio vettore centro geom lato- centro geom lato illuminato"
  If4/1 -> If Action Subsystem2/Action
  If Action Subsystem2/1(r_cface_cluce_yneg_z_neg) -> Merge3/1
  If3/1 -> If Action Subsystem1/Action
  [A_vect] -> If Action Subsystem/1(Areas_vect)
  Merge1/1 -> Add2/3  "raggio vettore centro geom lato- centro geom lato illuminato"
  If Action Subsystem4/1(r_cface_cluce_zneg_y_pos) -> Merge1/1
  Merge/1 -> Add2/2  "raggio vettore centro geom lato- centro geom lato illuminato"
  If Action Subsystem/1(r_cface_cluce_yz_pos) -> Merge/1
  If1/2 -> If Action Subsystem8/Action
  S_B/1 -> Reshape1/1
  Reshape1/1 -> Demux1/1
  Demux1/2 -> If2/2, If3/2, If4/2, If1/2  "S_B_y"
  If2/1 -> If Action Subsystem4/Action
  If1/1 -> If Action Subsystem/Action
  Demux1/3 -> If4/1, If3/1, If2/1, If1/1  "S_B_z"
  creating distance between cm MB and centro geom lato/1(Out1) -> Add2/1
  Demux1/1 -> Terminator1/1  "S_B_x"
  MB/1 -> [MB]
  [MB] -> If Action Subsystem/2(MB)
  [MB] -> If Action Subsystem4/2(MB)
  [MB] -> If Action Subsystem1/2(MB)
  [MB] -> If Action Subsystem2/2(MB)
  If Action Subsystem8/1(Out1) -> Merge/2
  If2/2 -> If Action Subsystem3/Action
  If3/2 -> If Action Subsystem5/Action
  If4/2 -> If Action Subsystem6/Action
  If Action Subsystem3/1(Out1) -> Merge1/2
  If Action Subsystem1/1(r_cface_cluce_yneg_z_pos) -> Merge2/1
  If Action Subsystem5/1(Out1) -> Merge2/2
  Merge2/1 -> Add2/4  "raggio vettore centro geom lato- centro geom lato illuminato"
  If Action Subsystem6/1(Out1) -> Merge3/2
  [MB] -> creating distance between cm MB and centro geom lato/1(MB)

== system Quaternions_Method_merge_1/Enviroment/Solar Radiation Perturbation/Sum forces/determine highlighted area/creazione della matrice che ha per colonne i vettori distanza tra il CM del MB e i centri geom delle aree illuminate dal sole /creazione raggi vettore tra CM MB e centro facce illuminate della faccia che ha come normale l'asse j ==
  S_B : Inport
  MB : Inport  Port=2
  Add2 : Sum  Inputs=+|+|+|+|+
  Demux1 : Demux  Outputs=3
  If Action Subsystem : Subsystem  TreatAsAtomicUnit=on
  If Action Subsystem1 : Subsystem  TreatAsAtomicUnit=on
  If Action Subsystem2 : Subsystem  TreatAsAtomicUnit=on
  If Action Subsystem3 : Subsystem  TreatAsAtomicUnit=on
  If Action Subsystem4 : Subsystem  TreatAsAtomicUnit=on
  If Action Subsystem5 : Subsystem  TreatAsAtomicUnit=on
  If Action Subsystem6 : Subsystem  TreatAsAtomicUnit=on
  If Action Subsystem7 : Subsystem  TreatAsAtomicUnit=on
  If1 : If  NumInputs=2  IfExpression=u1>0 & u2>0
  If2 : If  NumInputs=2  IfExpression=u1<0 & u2>0
  If3 : If  NumInputs=2  IfExpression=u1>0 & u2<0
  If4 : If  NumInputs=2  IfExpression=u1<0 & u2<0
  Merge{,1..3} (4 alike) : Merge
  Reshape1 : Reshape  OutputDimensionality=Column vector (2-D)
  Terminator1 : Terminator
  creating distance between cm MB and centro geom lato1 : Subsystem
  Out1 : Outport
  wires:
  Demux1/2 -> Terminator1/1
  creating distance between cm MB and centro geom lato1/1(Out1) -> Add2/1
  If1/1 -> If Action Subsystem/Action
  If2/1 -> If Action Subsystem1/Action
  Reshape1/1 -> Demux1/1
  S_B/1 -> Reshape1/1
  If Action Subsystem/1(r_cface_cluce_xz_pos) -> Merge/1
  Merge/1 -> Add2/2  "raggio vettore centro geom lato- centro geom lato illuminato"
  If Action Subsystem1/1(r_cface_cluce_x_pos_z_neg) -> Merge1/1
  Merge1/1 -> Add2/3  "raggio vettore centro geom lato- centro geom lato illuminato"
  [A_vect] -> If Action Subsystem/1(Areas_vect)
  Merge2/1 -> Add2/4  "raggio vettore centro geom lato- centro geom lato illuminato"
  If3/1 -> If Action Subsystem2/Action
  If Action Subsystem3/1(r_cface_cluce_x_neg_z_neg) -> Merge3/1
  If4/1 -> If Action Subsystem3/Action
  Merge3/1 -> Add2/5  "raggio vettore centro geom lato- centro geom lato illuminato"
  Add2/1 -> Out1/1
  [A_vect] -> If Action Subsystem1/1(Areas_vect)
  [A_vect] -> If Action Subsystem2/1(Areas_vect)
  [A_vect] -> If Action Subsystem3/1(Areas_vect)
  Demux1/3 -> If4/1, If3/1, If2/1, If1/1  "S_B_z"
  Demux1/1 -> If1/2, If4/2, If3/2, If2/2  "S_B_x"
  MB/1 -> [MB]
  [MB] -> If Action Subsystem/2(MB)
  [MB] -> If Action Subsystem1/2(MB)
  [MB] -> If Action Subsystem2/2(MB)
  [MB] -> If Action Subsystem3/2(MB)
  If1/2 -> If Action Subsystem5/Action
  If2/2 -> If Action Subsystem4/Action
  If3/2 -> If Action Subsystem6/Action
  If4/2 -> If Action Subsystem7/Action
  If Action Subsystem5/1(Out1) -> Merge/2
  If Action Subsystem4/1(Out1) -> Merge1/2
  If Action Subsystem2/1(r_cface_cluce_x_neg_z_pos) -> Merge2/1
  If Action Subsystem6/1(Out1) -> Merge2/2
  If Action Subsystem7/1(Out1) -> Merge3/2
  [MB] -> creating distance between cm MB and centro geom lato1/1(MB)

== system Quaternions_Method_merge_1/Enviroment/Solar Radiation Perturbation/Sum forces/determine highlighted area/creazione della matrice che ha per colonne i vettori distanza tra il CM del MB e i centri geom delle aree illuminate dal sole /creazione raggi vettore tra CM MB e centro facce illuminate della faccia che ha come normale l'asse k ==
  S_B : Inport
  MB : Inport  Port=2
  Add2 : Sum  Inputs=+|+|+|+|+
  Demux1 : Demux  Outputs=3
  If Action Subsystem : Subsystem  TreatAsAtomicUnit=on
  If Action Subsystem1 : Subsystem  TreatAsAtomicUnit=on
  If Action Subsystem2 : Subsystem  TreatAsAtomicUnit=on
  If Action Subsystem3 : Subsystem  TreatAsAtomicUnit=on
  If Action Subsystem4 : Subsystem  TreatAsAtomicUnit=on
  If Action Subsystem5 : Subsystem  TreatAsAtomicUnit=on
  If Action Subsystem6 : Subsystem  TreatAsAtomicUnit=on
  If Action Subsystem7 : Subsystem  TreatAsAtomicUnit=on
  If1 : If  NumInputs=2  IfExpression=u1>0 & u2>0
  If2 : If  NumInputs=2  IfExpression=u1<0 & u2>0
  If3 : If  NumInputs=2  IfExpression=u1>0 & u2<0
  If4 : If  NumInputs=2  IfExpression=u1<0 & u2<0
  Merge{,1..3} (4 alike) : Merge
  Reshape1 : Reshape  OutputDimensionality=Column vector (2-D)
  Terminator1 : Terminator
  creating distance between cm MB and centro geom lato1 : Subsystem
  Out1 : Outport
  wires:
  Demux1/3 -> Terminator1/1
  Demux1/1 -> If1/1, If4/1, If3/1, If2/1  "S_B_x"
  If1/1 -> If Action Subsystem/Action
  If2/1 -> If Action Subsystem4/Action
  Demux1/2 -> If4/2, If3/2, If2/2, If1/2  "S_B_y"
  Reshape1/1 -> Demux1/1
  S_B/1 -> Reshape1/1
  If1/2 -> If Action Subsystem5/Action
  Merge/1 -> Add2/2  "raggio vettore centro geom lato- centro geom lato illuminato"
  Merge1/1 -> Add2/3  "raggio vettore centro geom lato- centro geom lato illuminato"
  [A_vect] -> If Action Subsystem/1(Areas_vect)
  Merge2/1 -> Add2/4  "raggio vettore centro geom lato- centro geom lato illuminato"
  If3/2 -> If Action Subsystem6/Action
  If Action Subsystem1/1(r_cface_cluce_xpos_y_neg) -> Merge2/1
  If3/1 -> If Action Subsystem1/Action
  If4/2 -> If Action Subsystem7/Action
  If4/1 -> If Action Subsystem2/Action
  Merge3/1 -> Add2/5  "raggio vettore centro geom lato- centro geom lato illuminato"
  Add2/1 -> Out1/1
  [A_vect] -> If Action Subsystem4/1(Areas_vect)
  [A_vect] -> If Action Subsystem1/1(Areas_vect)
  [A_vect] -> If Action Subsystem2/1(Areas_vect)
  MB/1 -> [MB]
  [MB] -> If Action Subsystem/2(MB)
  [MB] -> If Action Subsystem4/2(MB1)
  [MB] -> If Action Subsystem1/2(MB)
  [MB] -> If Action Subsystem2/2(MB1)
  If2/2 -> If Action Subsystem3/Action
  If Action Subsystem/1(r_cface_cluce_xy_pos) -> Merge/1
  If Action Subsystem5/1(Out1) -> Merge/2
  If Action Subsystem4/1(r_cface_cluce_xneg_y_pos) -> Merge1/1
  If Action Subsystem3/1(Out1) -> Merge1/2
  If Action Subsystem6/1(Out1) -> Merge2/2
  If Action Subsystem2/1(r_cface_cluce_xneg_y_neg) -> Merge3/1
  If Action Subsystem7/1(Out1) -> Merge3/2
  [MB] -> creating distance between cm MB and centro geom lato1/1(MB)
  creating distance between cm MB and centro geom lato1/1(Out1) -> Add2/1

== system Quaternions_Method_merge_1/Enviroment/Solar Radiation Perturbation/Sum forces/determine highlighted area/creazione della matrice che ha per colonne i vettori distanza tra il CM del MB e i centri geom delle aree illuminate dal sole /creazione raggi vettore tra CM MB e centro facce illuminate della faccia che ha come normale l'asse i/If Action Subsystem ==
  Areas_vect : Inport
  MB : Inport  Port=2
  Action Port : ActionPort  ActionPortLabel=if(u1>0 & u2>0)
  Add : Sum  Inputs=+|-
  Add1 : Sum  Inputs=+|-
  Add2 : Sum
  Demux : Demux  Outputs=3
  Demux2 : Demux
  Divide : Product  Inputs=*/
  Divide1 : Product  Inputs=*/
  Gain{,1..3} (4 alike) : Gain  Gain=1/2
  Ground : Ground
  Ground1 : Ground
  Mux : Mux  Inputs=3
  Mux1 : Mux  Inputs=3
  Reshape : Reshape  OutputDimensionality=Column vector (2-D)
  Reshape2 : Reshape  OutputDimensionality=Column vector (2-D)
  Reshape3 : Reshape  OutputDimensionality=Column vector (2-D)
  Terminator{1..2,8..9} (4 alike) : Terminator
  r_cface_cluce_yz_pos : Outport
  wires:
  Demux/2 -> Terminator8/1
  Demux/3 -> Terminator9/1
  Add2/1 -> r_cface_cluce_yz_pos/1
  Reshape3/1 -> Add2/2
  Reshape2/1 -> Add2/1
  [h_MB] -> Gain2/1
  Divide1/1 -> Gain3/1
  Gain2/1 -> Add1/1
  Gain3/1 -> Add1/2
  Ground/1 -> Mux1/2, Mux1/1
  Mux1/1 -> Reshape3/1  "raggio vettore che collega il centro geom della faccia con il centro geom della faccia illuminata dal sole lungo k"
  [b_MB] -> Divide1/2
  Reshape/1 -> Demux/1
  Ground1/1 -> Mux/3, Mux/1
  Areas_vect/1 -> Reshape/1
  [h_MB] -> Divide/2
  Gain/1 -> Add/1
  [b_MB] -> Gain/1
  Gain1/1 -> Add/2
  Mux/1 -> Reshape2/1  "raggio vettore che collega il centro geom della faccia con il centro geom della faccia illuminata dal sole lungo j"
  Divide/1 -> Gain1/1
  Demux/1 -> Divide1/1, Divide/1
  Add/1 -> Mux/2
  Add1/1 -> Mux1/3
  Demux2/1 -> Terminator2/1
  Demux2/2 -> Terminator1/1
  MB/1 -> Demux2/1
  Demux2/3 -> [b_MB]
  Demux2/4 -> [h_MB]

== system Quaternions_Method_merge_1/Enviroment/Solar Radiation Perturbation/Sum forces/determine highlighted area/creazione della matrice che ha per colonne i vettori distanza tra il CM del MB e i centri geom delle aree illuminate dal sole /creazione raggi vettore tra CM MB e centro facce illuminate della faccia che ha come normale l'asse i/If Action Subsystem1 ==
  Areas_vect : Inport
  MB : Inport  Port=2
  Action Port : ActionPort  ActionPortLabel=if(u1>0 & u2<0)
  Add : Sum  Inputs=+|-
  Add1 : Sum  Inputs=+|-
  Add2 : Sum
  Demux : Demux  Outputs=3
  Demux2 : Demux
  Divide : Product  Inputs=*/
  Divide1 : Product  Inputs=*/
  Gain{,1..3} (4 alike) : Gain  Gain=1/2
  Gain4 : Gain  Gain=-1
  Ground : Ground
  Ground1 : Ground
  Mux : Mux  Inputs=3
  Mux1 : Mux  Inputs=3
  Reshape : Reshape  OutputDimensionality=Column vector (2-D)
  Reshape2 : Reshape  OutputDimensionality=Column vector (2-D)
  Reshape3 : Reshape  OutputDimensionality=Column vector (2-D)
  Terminator{1..2,8..9} (4 alike) : Terminator
  r_cface_cluce_yneg_z_pos : Outport
  wires:
  Add1/1 -> Mux1/3
  Demux/1 -> Divide/1, Divide1/1
  Divide/1 -> Gain1/1
  Mux/1 -> Reshape2/1  "raggio vettore che collega il centro geom della faccia con il centro geom della faccia illuminata dal sole lungo -j"
  Gain1/1 -> Add/2
  [b_MB] -> Gain/1
  Gain/1 -> Add/1
  [h_MB] -> Divide/2
  Areas_vect/1 -> Reshape/1
  Ground1/1 -> Mux/1, Mux/3
  Reshape/1 -> Demux/1
  [b_MB] -> Divide1/2
  Mux1/1 -> Reshape3/1  "raggio vettore che collega il centro geom della faccia con il centro geom della faccia illuminata dal sole lungo k"
  Ground/1 -> Mux1/1, Mux1/2
  Gain3/1 -> Add1/2
  Gain2/1 -> Add1/1
  Divide1/1 -> Gain3/1
  [h_MB] -> Gain2/1
  Reshape2/1 -> Add2/1
  Reshape3/1 -> Add2/2
  Add2/1 -> r_cface_cluce_yneg_z_pos/1
  Demux/3 -> Terminator9/1
  Demux/2 -> Terminator8/1
  Add/1 -> Gain4/1
  Gain4/1 -> Mux/2
  Demux2/1 -> Terminator2/1
  Demux2/2 -> Terminator1/1
  MB/1 -> Demux2/1
  Demux2/3 -> [b_MB]
  Demux2/4 -> [h_MB]

== system Quaternions_Method_merge_1/Enviroment/Solar Radiation Perturbation/Sum forces/determine highlighted area/creazione della matrice che ha per colonne i vettori distanza tra il CM del MB e i centri geom delle aree illuminate dal sole /creazione raggi vettore tra CM MB e centro facce illuminate della faccia che ha come normale l'asse i/If Action Subsystem2 ==
  Areas_vect : Inport
  MB : Inport  Port=2
  Action Port : ActionPort  ActionPortLabel=if(u1<0 & u2<0)
  Add : Sum  Inputs=+|-
  Add1 : Sum  Inputs=+|-
  Add2 : Sum
  Demux : Demux  Outputs=3
  Demux2 : Demux
  Divide : Product  Inputs=*/
  Divide1 : Product  Inputs=*/
  Gain{,1..3} (4 alike) : Gain  Gain=1/2
  Gain4 : Gain  Gain=-1
  Gain5 : Gain  Gain=-1
  Ground : Ground
  Ground1 : Ground
  Mux : Mux  Inputs=3
  Mux1 : Mux  Inputs=3
  Reshape : Reshape  OutputDimensionality=Column vector (2-D)
  Reshape2 : Reshape  OutputDimensionality=Column vector (2-D)
  Reshape3 : Reshape  OutputDimensionality=Column vector (2-D)
  Terminator{1..2,8..9} (4 alike) : Terminator
  r_cface_cluce_yneg_z_neg : Outport
  wires:
  Gain4/1 -> Mux/2
  Add/1 -> Gain4/1
  Demux/2 -> Terminator8/1
  Demux/3 -> Terminator9/1
  Add2/1 -> r_cface_cluce_yneg_z_neg/1
  Reshape3/1 -> Add2/2
  Reshape2/1 -> Add2/1
  [h_MB] -> Gain2/1
  Divide1/1 -> Gain3/1
  Gain2/1 -> Add1/1
  Gain3/1 -> Add1/2
  Ground/1 -> Mux1/2, Mux1/1
  Mux1/1 -> Reshape3/1  "raggio vettore che collega il centro geom della faccia con il centro geom della faccia illuminata dal sole lungo -k"
  [b_MB] -> Divide1/2
  Reshape/1 -> Demux/1
  Ground1/1 -> Mux/3, Mux/1
  Areas_vect/1 -> Reshape/1
  [h_MB] -> Divide/2
  Gain/1 -> Add/1
  [b_MB] -> Gain/1
  Gain1/1 -> Add/2
  Mux/1 -> Reshape2/1  "raggio vettore che collega il centro geom della faccia con il centro geom della faccia illuminata dal sole lungo -j"
  Divide/1 -> Gain1/1
  Demux/1 -> Divide1/1, Divide/1
  Gain5/1 -> Mux1/3
  Add1/1 -> Gain5/1
  Demux2/1 -> Terminator2/1
  Demux2/2 -> Terminator1/1
  MB/1 -> Demux2/1
  Demux2/3 -> [b_MB]
  Demux2/4 -> [h_MB]

== system Quaternions_Method_merge_1/Enviroment/Solar Radiation Perturbation/Sum forces/determine highlighted area/creazione della matrice che ha per colonne i vettori distanza tra il CM del MB e i centri geom delle aree illuminate dal sole /creazione raggi vettore tra CM MB e centro facce illuminate della faccia che ha come normale l'asse i/If Action Subsystem3 ==
  Action Port : ActionPort  ActionPortLabel=else
  Constant : Constant  Value=[0;0;0]
  Out1 : Outport
  wires:
  Constant/1 -> Out1/1
